simulink library "Du_Gimbal_LIB"  (R2024b)
settings: Solver=VariableStepAuto  StartTime=0.0  StopTime=10.0  RelTol=1e-3
undefined symbols (not defined in the file): Continuous, DiscIntNeverNeededParam, params, Time, Ts
libraries: arduinolib x12, fl_lib x11, nesl_utility x7, $bdroot x5, simulink x4, simulink_extras x3, MISSILE_GUIDANCE_LIB2 x3, dspstat3 x3, hdlsllib x2, ctrlSharedLib x1, ee_lib x1, arduinosensorlib x1
settings Model: Creator=leoni  LastModifiedBy=leoni

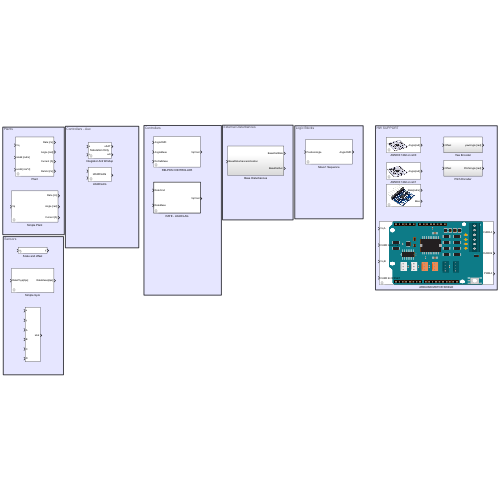
[thumbnail: Simulink's stored preview of the top-level diagram]
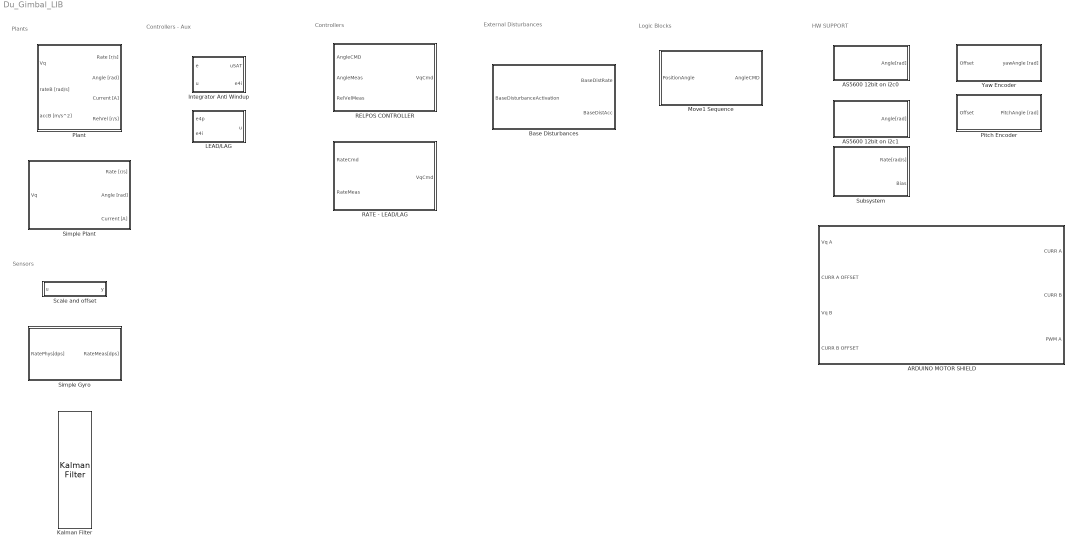
== system Du_Gimbal_LIB ==
  note: HW SUPPORT
  note: Sensors
  note: Logic Blocks
  note: Controllers
  note: Controllers - Aux
  note: Plants
  note: External Disturbances
  ARDUINO MOTOR SHIELD : Subsystem  mask{ts=1/1000, VqMax=0.85, motAdirReverse=off, motBdirReverse=off}
      mask prompts: ts "Sample Time [s]"; VqMax "Vq max."; motAdirReverse "motor A Current direction Reversed ?"; motBdirReverse "motor B Current direction Reversed ?"
      mask Display: image('arduino_motor_shield_sized_1.svg');
  AS5600 12bit on i2c0 : Subsystem  mask{deviceAddress=0x36, angleRegAddress=0x0C, ts=0.01}
      mask prompts: deviceAddress "AS 5600 Address"; angleRegAddress "Angle register"; ts "Sample Time [s]"
      mask Display: image('AS5600_ENC.png');
  AS5600 12bit on i2c1 : Subsystem  mask{deviceAddress=0x36, angleRegAddress=0x0C, ts=0.01}
      mask prompts: deviceAddress "AS 5600 Address"; angleRegAddress "Angle register"; ts "Read Time Step"
      mask Display: image('AS5600_ENC.png');
  Base Disturbances : Subsystem
  Integrator Anti Windup : Subsystem  mask{clampingOn=off, satLimit=0}
      mask prompts: clampingOn "AntiWindup Active"; satLimit "Saturation Limit"
      mask Display:
      | p = Simulink.Mask.get(gcb);
      | param = p.getParameter('clampingOn');
      | clampingOn = param.Value;
      | if contains(clampingOn,'on')
      | disp('Integrator Clamping Active');
      | else
      | disp('Saturation Only');
      | end
  Kalman Filter : ctrlSharedLib/Kalman Filter  TimeDomain=Continuous-Time  UseCurrentEstimator=on  ModelSource=Input port  ModelSourceVariable=ss(0.95,1,1,0,1)  A=0.95  B=1  C=1  D=0  NumberOfStates=1  NumberOfInputs=1  NumberOfOutputs=1  InitialEstimateSource=Dialog  X0=0  P0=10  UseK=off  UseGH=off  NumberOfProcessNoiseInputs=1  G=1  TimeInvariantG=on  H=0  TimeInvariantH=on  Q=0.05  TimeInvariantQ=on  R=1  TimeInvariantR=on  N=0  TimeInvariantN=on  AddInputPort=on  AddEnablePort=off  OutputEstimatedY=off  OutputP=off  Ts=-1
  LEAD/LAG : Subsystem  mask{isPiFlag=0, Kc=0, tau_N=0, tau_D=1.0, Ts=0}
      mask prompts: isPiFlag "is PI ?"; Kc "Controller Gain"; tau_N "Numerator Time Constant [s]"; tau_D "Denominator time Constant [s]"; Ts "Sampling Time [s]"
      mask Callback isPiFlag:
      | p = Simulink.Mask.get(gcb);
      |     param = p.getParameter('isPiFlag');
      |     slave = p.getParameter('tau_D');
      |     isPI = param.Value;
      |     if contains(isPI,'1')
      |         slave.Value = '1.0';
      |         slave.Visible = 'off';
      |     else
      |         slave.Visible = 'on';
      |     end
      mask Display:
      | p = Simulink.Mask.get(gcb);
      | param = p.getParameter('isPiFlag');
      | isPi = param.Value;
      | if contains(isPi,'1')
      | disp('PI Controller');
      | else
      | disp('LEAD/LAG');
      | end
  Move1 Sequence : Subsystem  mask{theta_dot_cmd=5, theta_travel=16, t_start=2, t_at_limit=0.5, theta_delta=1.0}
      mask prompts: theta_dot_cmd "Motion Speed [deg/s]"; theta_travel "Single Side Angle [deg]"; t_start "Start Motion Time [s]"; t_at_limit "Limit Idle Time [s]"; theta_delta "Limit Proximity Value [deg]"
      mask DialogControl ParameterGroupVar Prompt: Move1 Generator
  Pitch Encoder : Subsystem
  Plant : Subsystem  mask{L_m=1.2e-3, R_m=6.9, Kt=0.0116, V_bus=6.0, J_m=3.2e-7, J_L=200e-6, limit_DEG=17, T_r=1.8e-3, K_spr=25e-3, UNB_mag=300e-6, UNB_pos=deg2rad(45)}
      mask prompts: L_m "Inductance [H]"; R_m "Resistance [Ohm]"; Kt "Torque Constant [Nm/A]"; V_bus "Vbus [V]"; J_m "Motor Rotor Inertia [kg m^2]"; J_L "Load Inertia [kg m^2]"; limit_DEG "Travel Limit [deg]"; T_r "Friction Torque [Nm]"; K_spr "Spring Constant [Nm/Rad]"; UNB_mag "Unbalance Mag. [kg*m]"; UNB_pos "Unbalance Angle [rad]"
      mask DialogControl ParameterGroupVar Prompt: Motor Parameters
      mask DialogControl Container3 Prompt: Load Properties
      mask DialogControl Container4 Prompt: Disturbances Properties
  RATE - LEAD/LAG : Subsystem  TreatAsAtomicUnit=on  SystemSampleTime=Ts  mask{lagParams=params.LAG, leadParams=params.LEAD, VqRatioFromMAX=0.95, VqMAX=1.0}
      mask prompts: lagParams "LAG Controller Parameters"; leadParams "LEAD Controller Parameters"; VqRatioFromMAX "Vq Clamping Ratio from MAX."; VqMAX "Vq Max. CMD"
      mask DialogControl ParameterGroupVar Prompt: Controllers
      mask DialogControl Container3 Prompt: Saturations
  RELPOS CONTROLLER : Subsystem  mask{Kp=25, Kv=2.5, Vq_sat=0.95}
      mask prompts: Kp "Angle Error Gain"; Kv "Vel Error Gain"; Vq_sat "Max. Vq Cmd."
      mask DialogControl ParameterGroupVar Prompt: RELPOS CASCADE
  Scale and offset : Subsystem  mask{scale=0, offset=0}
  Simple Gyro : Subsystem  mask{scaleFactor=params.GYRO.SF_proc, a2dSens=params.GYRO.a2dSens, gyrosMA=params.GYRO.gyrosMA_proc, bias=params.GYRO.bias, biasInstability=params.GYRO.biasInstability, gSens=params.GYRO.gSens, noiseDensity=params.GYRO.noiseDensity, friqFIlter=params.GYRO.freqFilter, zetaFilter=params.GYRO.zetaFilter, dataRate=params.GYRO.dataRate, rngSeed=0}
      mask prompts: scaleFactor "Scale Factor [%]"; a2dSens "Sensetivity Scale Factor [LSB/dps]"; gyrosMA "Cross Axis Sensetivity [%]"; bias "Bias [deg/s]"; biasInstability "Time Drift [deg/s/s]"; gSens "Linear Acceleration Sensetivity"; noiseDensity "Noise Denisty [dps/sqrt_Hz]"; friqFIlter "Filter Bandwith [Hz]"; zetaFilter "Filter Zeta"; dataRate "Data Rate [Hz]"; rngSeed "RNG SEED"
      mask init:
      | rng(rngSeed);
      |     randFactors = rand(7,1)*2-1;
      mask DialogControl ParameterGroupVar Prompt: GYROSCOPE SENSETIVITY
      mask DialogControl Container4 Prompt: Gyroscope Zero Rate output
      mask DialogControl Container5 Prompt: Gyroscope Noise Performance
      mask DialogControl Container3 Prompt: FIlter Properties
      mask DialogControl Container6 Prompt: DATA RATE
  Simple Plant : Subsystem  mask{plantParams=params.PLANT}
      mask prompts: plantParams "Plant And Actuator Params"
  Subsystem : Subsystem  mask{ts=0, tInit=0}
      mask prompts: ts "Sampling Time [s]"; tInit "Initialization Time [s]"
      mask Display: image('MPU6050_ICON.svg');
  Yaw Encoder : Subsystem

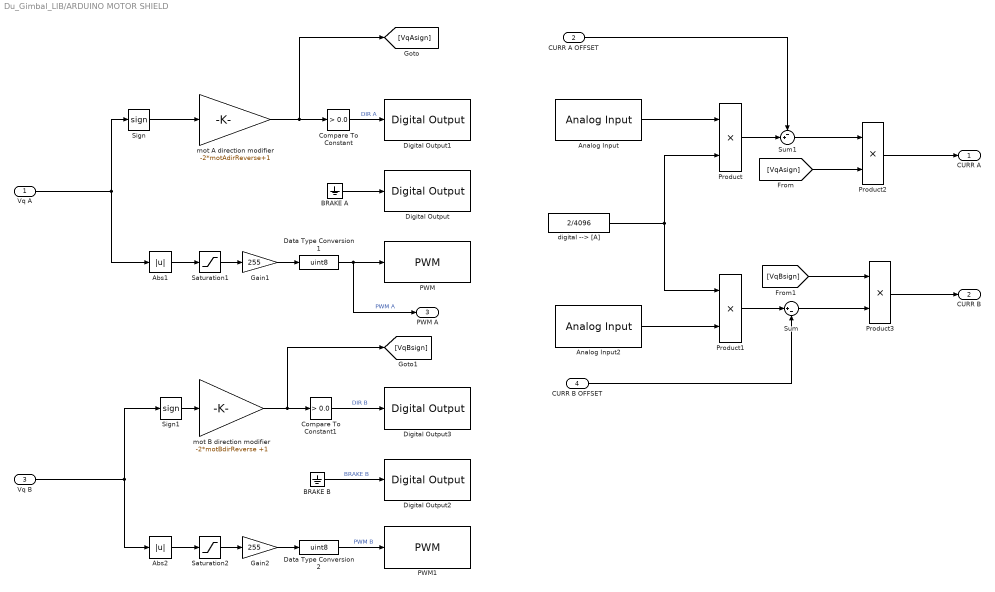
== system Du_Gimbal_LIB/ARDUINO MOTOR SHIELD ==
  Vq A : Inport
  CURR A OFFSET : Inport  Port=2
  Vq B : Inport  Port=3
  CURR B OFFSET : Inport  Port=4
  Abs1 : Abs  SaturateOnIntegerOverflow=off
  Abs2 : Abs  SaturateOnIntegerOverflow=off
  Analog Input : arduinolib/Analog Input  pinNumber=0  ReadResultsOnly=off  ConversionTriggerSource=Software  ExternalTriggerType=uint32( 0 )  OutputDataType=uint16  EnableConversionCompleteNotify=off  EnableOuputStatus=off  SampleTime=ts  blockPlatform=arduino
      settings: SourceProductName=Common
  Analog Input2 : arduinolib/Analog Input  pinNumber=1  ReadResultsOnly=off  ConversionTriggerSource=Software  ExternalTriggerType=uint32( 0 )  OutputDataType=uint16  EnableConversionCompleteNotify=off  EnableOuputStatus=off  SampleTime=ts  blockPlatform=arduino
      settings: SourceProductName=Common
  BRAKE A : Ground
  BRAKE B : Ground
  Compare To Constant : simulink/Logic and Bit Operations/Compare To Constant  relop=>  const=0.0  OutDataTypeStr=boolean
  Compare To Constant1 : simulink/Logic and Bit Operations/Compare To Constant  relop=>  const=0.0  OutDataTypeStr=boolean
  Data Type Conversion1 : DataTypeConversion  OutDataTypeStr=uint8  SaturateOnIntegerOverflow=off  RndMeth=Floor
  Data Type Conversion2 : DataTypeConversion  OutDataTypeStr=uint8  SaturateOnIntegerOverflow=off  RndMeth=Floor
  Digital Output : arduinolib/Digital Output  pinNumber=9  Direction=output  blockPlatform=arduino
      settings: SourceProductName=Common
  Digital Output1 : arduinolib/Digital Output  pinNumber=12  Direction=output  blockPlatform=arduino
      settings: SourceProductName=Common
  Digital Output2 : arduinolib/Digital Output  pinNumber=8  Direction=output  blockPlatform=arduino
      settings: SourceProductName=Common
  Digital Output3 : arduinolib/Digital Output  pinNumber=13  Direction=output  blockPlatform=arduino
      settings: SourceProductName=Common
  Gain1 : Gain  Gain=255  OutDataTypeStr=uint16
  Gain2 : Gain  Gain=255  OutDataTypeStr=uint16
  PWM : arduinolib/PWM  pinNumber=3  frequencyType=Specify  desiredFrequency=50000  achievableFrequency=490.2
      settings: SourceProductName=Common
  PWM1 : arduinolib/PWM  pinNumber=11  frequencyType=Specify  desiredFrequency=50000  achievableFrequency=490.2
      settings: SourceProductName=Common
  Product{,1..3} (4 alike) : Product
  Saturation1 : Saturate  UpperLimit=VqMax  LowerLimit=0
  Saturation2 : Saturate  UpperLimit=VqMax  LowerLimit=0
  Sign : Signum
  Sign1 : Signum
  Sum : Sum  Inputs=|+-
  Sum1 : Sum  Inputs=-+|
  digital --> [A] : Constant  Value=2/4096
  mot A direction modifier : Gain  Gain=-2*motAdirReverse+1
  mot B direction modifier : Gain  Gain=-2*motBdirReverse +1
  CURR A : Outport
  CURR B : Outport  Port=2
  PWM A : Outport  Port=3
  wires:
  BRAKE B/1 -> Digital Output2/1  "BRAKE B"
  Data Type Conversion2/1 -> PWM1/1  "PWM B"
  BRAKE A/1 -> Digital Output/1
  Data Type Conversion1/1 -> PWM A/1, PWM/1  "PWM A"
  Analog Input2/1 -> Product1/2
  Product/1 -> Sum1/2
  Product1/1 -> Sum/1
  digital --> [A]/1 -> Product/2, Product1/1
  Analog Input/1 -> Product/1
  CURR A OFFSET/1 -> Sum1/1
  Sum1/1 -> Product2/1
  Sum/1 -> Product3/2
  CURR B OFFSET/1 -> Sum/2
  Vq A/1 -> Abs1/1, Sign/1
  Abs1/1 -> Saturation1/1
  Saturation1/1 -> Gain1/1
  Gain1/1 -> Data Type Conversion1/1
  Sign1/1 -> mot B direction modifier/1
  Vq B/1 -> Sign1/1, Abs2/1
  Abs2/1 -> Saturation2/1
  Saturation2/1 -> Gain2/1
  Gain2/1 -> Data Type Conversion2/1
  Compare To Constant/1 -> Digital Output1/1  "DIR A"
  Compare To Constant1/1 -> Digital Output3/1  "DIR B"
  Product2/1 -> CURR A/1
  [VqAsign] -> Product2/2
  [VqBsign] -> Product3/1
  Product3/1 -> CURR B/1
  mot A direction modifier/1 -> [VqAsign], Compare To Constant/1
  mot B direction modifier/1 -> [VqBsign], Compare To Constant1/1
  Sign/1 -> mot A direction modifier/1

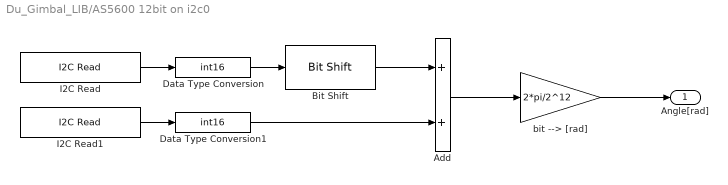
== system Du_Gimbal_LIB/AS5600 12bit on i2c0 ==
  Add : Sum
  Bit Shift : hdlsllib/Logic and Bit Operations/Bit Shift  mode=Shift Left Logical  N=8
  Data Type Conversion : DataTypeConversion  OutDataTypeStr=int16  SaturateOnIntegerOverflow=off  RndMeth=Floor
  Data Type Conversion1 : DataTypeConversion  OutDataTypeStr=int16  SaturateOnIntegerOverflow=off  RndMeth=Floor
  I2C Read : arduinolib/I2C Read  I2CModule=0  Mode=Master  SlaveAddress=deviceAddress  SlaveByteOrder=BigEndian  Direction=Receiver  RegisterAddressMode=on  RegisterAddress=angleRegAddress  SlaveDataType=uint8  DataLength=1  NoAck=off  RepeatedStart=off  OutputStatus=off  blockPlatform=ARDUINO  SampleTime=ts
      settings: SourceProductName=Common
  I2C Read1 : arduinolib/I2C Read  I2CModule=0  Mode=Master  SlaveAddress=deviceAddress  SlaveByteOrder=BigEndian  Direction=Receiver  RegisterAddressMode=on  RegisterAddress=angleRegAddress+1  SlaveDataType=uint8  DataLength=1  NoAck=off  RepeatedStart=off  OutputStatus=off  blockPlatform=ARDUINO  SampleTime=ts
      settings: SourceProductName=Common
  bit --> [rad] : Gain  Gain=2*pi/2^12
  Angle[rad] : Outport
  wires:
  Data Type Conversion1/1 -> Add/2
  Bit Shift/1 -> Add/1
  Data Type Conversion/1 -> Bit Shift/1
  I2C Read/1 -> Data Type Conversion/1
  I2C Read1/1 -> Data Type Conversion1/1
  Add/1 -> bit --> [rad]/1
  bit --> [rad]/1 -> Angle[rad]/1

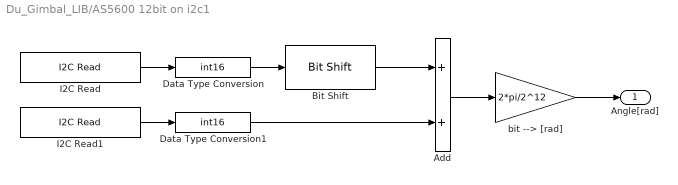
== system Du_Gimbal_LIB/AS5600 12bit on i2c1 ==
  Add : Sum
  Bit Shift : hdlsllib/Logic and Bit Operations/Bit Shift  mode=Shift Left Logical  N=8
  Data Type Conversion : DataTypeConversion  OutDataTypeStr=int16  SaturateOnIntegerOverflow=off  RndMeth=Floor
  Data Type Conversion1 : DataTypeConversion  OutDataTypeStr=int16  SaturateOnIntegerOverflow=off  RndMeth=Floor
  I2C Read : arduinolib/I2C Read  I2CModule=1  Mode=Master  SlaveAddress=deviceAddress  SlaveByteOrder=BigEndian  Direction=Receiver  RegisterAddressMode=on  RegisterAddress=angleRegAddress  SlaveDataType=uint8  DataLength=1  NoAck=off  RepeatedStart=off  OutputStatus=off  blockPlatform=ARDUINO  SampleTime=ts
      settings: SourceProductName=Common
  I2C Read1 : arduinolib/I2C Read  I2CModule=1  Mode=Master  SlaveAddress=deviceAddress  SlaveByteOrder=BigEndian  Direction=Receiver  RegisterAddressMode=on  RegisterAddress=angleRegAddress+1  SlaveDataType=uint8  DataLength=1  NoAck=off  RepeatedStart=off  OutputStatus=off  blockPlatform=ARDUINO  SampleTime=ts
      settings: SourceProductName=Common
  bit --> [rad] : Gain  Gain=2*pi/2^12
  Angle[rad] : Outport
  wires:
  Data Type Conversion1/1 -> Add/2
  Bit Shift/1 -> Add/1
  Data Type Conversion/1 -> Bit Shift/1
  I2C Read/1 -> Data Type Conversion/1
  I2C Read1/1 -> Data Type Conversion1/1
  Add/1 -> bit --> [rad]/1
  bit --> [rad]/1 -> Angle[rad]/1

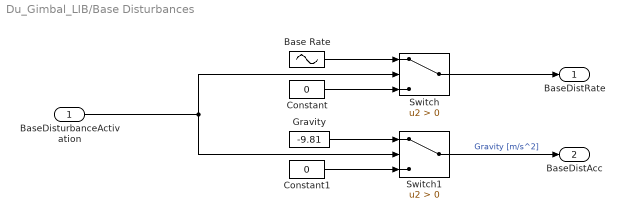
== system Du_Gimbal_LIB/Base Disturbances ==
  BaseDisturbanceActivation : Inport
  Base Rate : Sin  Amplitude=deg2rad(20)  Frequency=2*pi*2  SampleTime=0
  Constant : Constant  Value=0
  Constant1 : Constant  Value=0
  Gravity : Constant  Value=-9.81
  Switch : Switch  Criteria=u2 > Threshold  SaturateOnIntegerOverflow=off  InputSameDT=off
  Switch1 : Switch  Criteria=u2 > Threshold  SaturateOnIntegerOverflow=off  InputSameDT=off
  BaseDistRate : Outport
  BaseDistAcc : Outport  Port=2
  wires:
  BaseDisturbanceActivation/1 -> Switch1/2, Switch/2
  Constant/1 -> Switch/3
  Gravity/1 -> Switch1/1
  Base Rate/1 -> Switch/1
  Switch/1 -> BaseDistRate/1
  Constant1/1 -> Switch1/3
  Switch1/1 -> BaseDistAcc/1  "Gravity [m/s^2]"

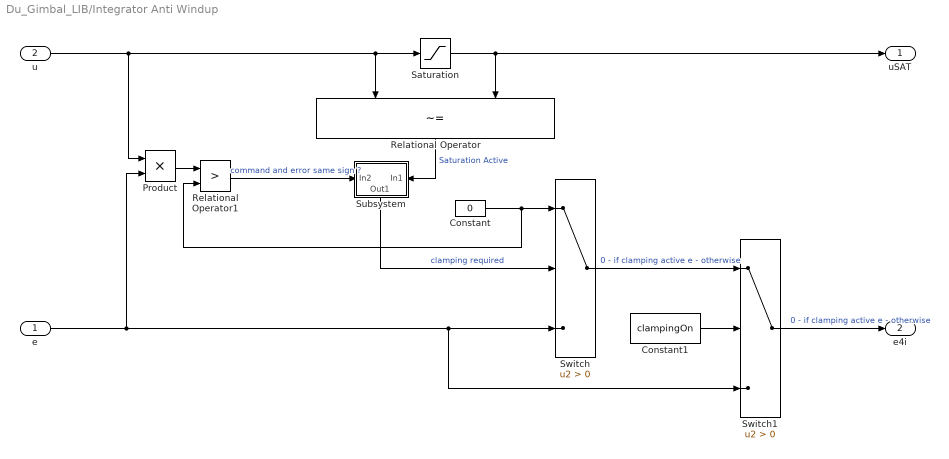
== system Du_Gimbal_LIB/Integrator Anti Windup ==
  e : Inport
  u : Inport  Port=2
  Constant : Constant  Value=0
  Constant1 : Constant  Value=clampingOn
  Product : Product
  Relational Operator : RelationalOperator  Operator=~=  OutDataTypeStr=boolean  RndMeth=Simplest  InputSameDT=off
  Relational Operator1 : RelationalOperator  Operator=>  OutDataTypeStr=boolean  RndMeth=Simplest  InputSameDT=off
  Saturation : Saturate  UpperLimit=satLimit  LowerLimit=-satLimit
  Subsystem : Subsystem
      settings: PortSchema="{\"entries\":[{\"content\":{\"sides\":[{\"content\":{},\"type\":\"ConnectorPlacement.EquallySpacedRectSide\",\"uuid\":\"a9aec0d1-7f20-4b23-b37e-cf2c45620145\"},{\"content\":{\"connectorIds\":[\"Out1\"],\"side\":\"RIGHT\"},\"type\":\"ConnectorPlacement.EquallySpacedRectSide\",\"uuid\":\"46d94b5a-ca40-426c-ab7c-6dcf988cef68\"},{\"content\":{\"connectorIds\":[\"In1\"],\"side\":\"TOP\"},\"type\":\"ConnectorPlacement.EquallySpacedRectSide\",\"uuid\":\"2dd56584-143a-41c5-aa39-bf48e1e5c5d9\"},{\"content\":{\"connectorIds\":[\"In2\"],\"side\":\"BOTTOM\"},\"type\":\"ConnectorPlacement.EquallySpacedRectSide\",\"uuid\":\"3500ab9b-abc5-4f65-b64c-eef04de61636\"}]},\"type\":\"ConnectorPlacement.EquallySpacedConnector\",\"uuid\":\"f9745eab-cd5d-404d-8705-919820576021\"}],\"packageUris\":[\"http://schema.mathworks.com/mf0/Connector/R2020b\"],\"version\":\"1.0\"}"
      mask Display: disp('AND');
  Switch : Switch  Criteria=u2 > Threshold  SaturateOnIntegerOverflow=off  InputSameDT=off
  Switch1 : Switch  Criteria=u2 > Threshold  SaturateOnIntegerOverflow=off  InputSameDT=off
  uSAT : Outport
  e4i : Outport  Port=2
  wires:
  e/1 -> Product/2, Switch1/3, Switch/3
  Subsystem/1(Out1) -> Switch/2  "clamping required"
  u/1 -> Product/1, Saturation/1, Relational Operator/1
  Saturation/1 -> uSAT/1, Relational Operator/2
  Relational Operator/1 -> Subsystem/2(In1)  "Saturation Active"
  Switch/1 -> Switch1/1  "0 - if clamping active e - otherwise"
  Constant/1 -> Relational Operator1/2, Switch/1
  Product/1 -> Relational Operator1/1
  Relational Operator1/1 -> Subsystem/1(In2)  "command and error same sign ?"
  Switch1/1 -> e4i/1  "0 - if clamping active e - otherwise"
  Constant1/1 -> Switch1/2

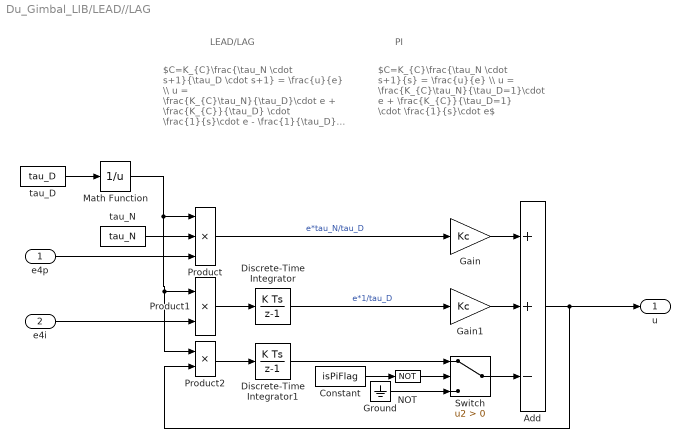
== system Du_Gimbal_LIB/LEAD//LAG ==
  note: LEAD/LAG
  note: $C=K_{C}\frac{\tau_N \cdot s+1}{\tau_D \cdot s+1} = \frac{u}{e} \\ u = \frac{K_{C}\tau_N}{\tau_D}\cdot e + \frac{K_{C}}{\tau_D} \cdot \frac{1}{s}\cdot e - \frac{1}{\tau_D} \cdot \frac{1}{s}\cdot u$
  note: PI
  note: $C=K_{C}\frac{\tau_N \cdot s+1}{s} = \frac{u}{e} \\ u = \frac{K_{C}\tau_N}{\tau_D=1}\cdot e + \frac{K_{C}}{\tau_D=1} \cdot \frac{1}{s}\cdot e$
  e4p : Inport
  e4i : Inport  Port=2
  Add : Sum  Inputs=++-
  Constant : Constant  Value=isPiFlag
  Discrete-Time Integrator : DiscreteIntegrator  SampleTime=Ts  ICPrevOutput=DiscIntNeverNeededParam  ICPrevScaledInput=DiscIntNeverNeededParam
  Discrete-Time Integrator1 : DiscreteIntegrator  SampleTime=Ts  ICPrevOutput=DiscIntNeverNeededParam  ICPrevScaledInput=DiscIntNeverNeededParam
  Gain : Gain  Gain=Kc
  Gain1 : Gain  Gain=Kc
  Ground : Ground
  Math Function : Math  Operator=reciprocal
  NOT : Logic  Operator=NOT  AllPortsSameDT=off  OutDataTypeStr=boolean
  Product : Product  Inputs=***
  Product1 : Product  Inputs=**
  Product2 : Product  Inputs=**
  Switch : Switch  Criteria=u2 > Threshold  SaturateOnIntegerOverflow=off  InputSameDT=off
  tau_D : Constant  Value=tau_D
  tau_N : Constant  Value=tau_N
  u : Outport
  wires:
  e4p/1 -> Product/3
  Add/1 -> Product2/2, u/1
  tau_D/1 -> Math Function/1
  Math Function/1 -> Product2/1, Product1/1, Product/1
  tau_N/1 -> Product/2
  Product/1 -> Gain/1  "e*tau_N/tau_D"
  Product1/1 -> Discrete-Time Integrator/1
  Discrete-Time Integrator/1 -> Gain1/1  "e*1/tau_D"
  Product2/1 -> Discrete-Time Integrator1/1
  Discrete-Time Integrator1/1 -> Switch/1
  e4i/1 -> Product1/2
  Gain/1 -> Add/1
  Gain1/1 -> Add/2
  Switch/1 -> Add/3
  Constant/1 -> NOT/1
  NOT/1 -> Switch/2
  Ground/1 -> Switch/3

== system Du_Gimbal_LIB/Move1 Sequence ==
  PositionAngle : Inport
  Degrees to Radians : simulink_extras/Transformations/Degrees to Radians
  MOVE1 LOGIC - Degrees : Stateflow chart  TreatAsAtomicUnit=on
  Radians to Degrees : simulink_extras/Transformations/Radians to Degrees
  Rate Limiter : RateLimiter  RisingSlewLimit=theta_dot_cmd  FallingSlewLimit=-theta_dot_cmd  SampleTimeMode=inherited
  AngleCMD : Outport
  wires:
  MOVE1 LOGIC - Degrees/1(PosCmd) -> Rate Limiter/1
  Degrees to Radians/1 -> AngleCMD/1
  Rate Limiter/1 -> Degrees to Radians/1
  PositionAngle/1 -> Radians to Degrees/1
  Radians to Degrees/1 -> MOVE1 LOGIC - Degrees/1(PosRtn)

== system Du_Gimbal_LIB/Pitch Encoder ==
  Offset : Inport
  AS5600 12bit on i2c1 : $bdroot/AS5600 12bit on i2c1  deviceAddress=0x36  angleRegAddress=0x0C  ts=0.01
  DirectionModifier : Gain  Gain=-1
  Sum : Sum  Inputs=|+-
  PitchAngle [rad] : Outport
  wires:
  Sum/1 -> DirectionModifier/1
  AS5600 12bit on i2c1/1 -> Sum/1
  Offset/1 -> Sum/2
  DirectionModifier/1 -> PitchAngle [rad]/1

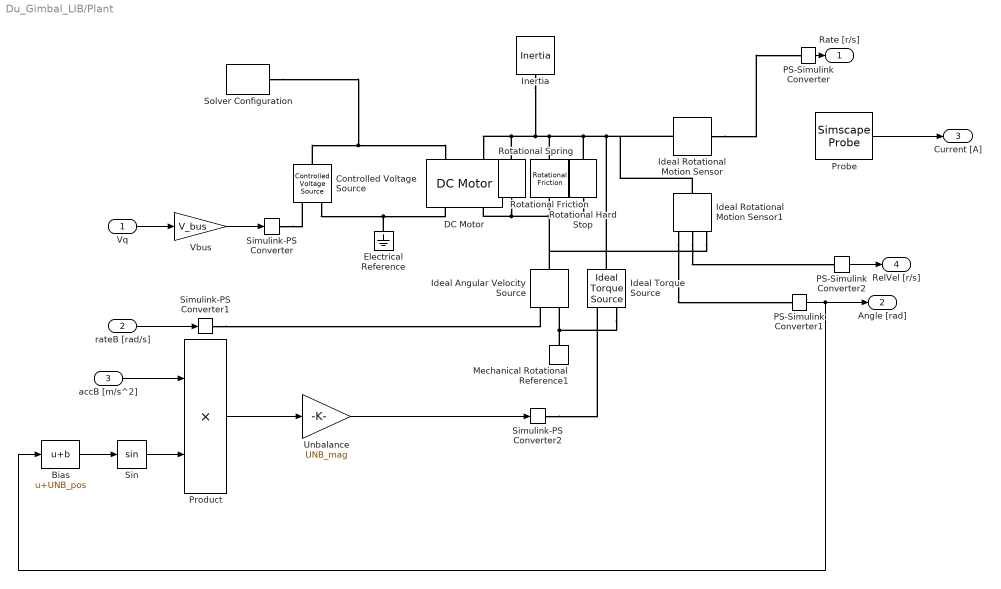
== system Du_Gimbal_LIB/Plant ==
  Vq : Inport
  rateB [rad/s] : Inport  Port=2
  accB [m/s^2] : Inport  Port=3
  Bias : Bias  Bias=UNB_pos  SaturateOnIntegerOverflow=off
  Controlled Voltage Source : fl_lib/Electrical/Electrical Sources/Controlled Voltage Source
  DC Motor : ee_lib/Electromechanical/Brushed Motors/DC Motor  field_option=ee.enum.field_option.pm  Rf=100 Ohm  Lf=1 H  Laf=0.15 H  If0=0 A  parameterization=ee.enum.dcparam_option.circuit_param  Ra=R_m Ohm  La=L_m H  emf_or_torque=ee.enum.emf_or_torque.kv  Kv=Kt V/(rad/s)  Ki=6.876e-4 N*m/A  T_stall=T_p N*m  w_max=w_NL rad/s  w_rated=15000 rpm  P_rated=0.08 W  V_rated=V_n V  lam_param=ee.enum.lam_param.damping  i_noload=0 A  V_i_noload=1.5 V  J=J_m kg*m^2  lam=0 N*m*s/rad  speed0=0 rpm  t_fault_armature=1 s  t_fault_field=1 s  fault_action=simscape.enum.assert.action.none  alpha=3.93e-3 1/K  Tmeas=25 degC  thermal_mass=100 J/K  initial_temperature=25 degC
  Electrical Reference : fl_lib/Electrical/Electrical Elements/Electrical Reference
  Ideal Angular Velocity Source : fl_lib/Mechanical/Mechanical Sources/Ideal Angular Velocity Source
  Ideal Rotational Motion Sensor : fl_lib/Mechanical/Mechanical Sensors/Ideal Rotational Motion Sensor  reference=foundation.enum.MeasurementReference.absolute  acceleration_port=false  velocity_port=true  position_port=false  wrap_angle=false  offset=0 deg
      settings: InternalSimscapePortConfiguration="{\"Bottom\":[],\"Left\":[{\"id\":\"R\",\"label\":\"R\",\"type\":\"foundation.mechanical.rotational.rotational\"}],\"Right\":[{\"id\":\"W\",\"label\":\"W\",\"type\":\"output\"}],\"Top\":[]}"
  Ideal Rotational Motion Sensor1 : fl_lib/Mechanical/Mechanical Sensors/Ideal Rotational Motion Sensor  reference=foundation.enum.MeasurementReference.difference  acceleration_port=false  velocity_port=true  position_port=true  wrap_angle=false  offset=0 rad
  Ideal Torque Source : fl_lib/Mechanical/Mechanical Sources/Ideal Torque Source
  Inertia : fl_lib/Mechanical/Rotational Elements/Inertia  inertia=J_L kg*m^2  num_ports=foundation.enum.numPorts2.one  w_specify=off  w_priority=High  w=0 rad/s  w_nominal_specify=off  w_nominal_value=1  w_nominal_unit=rad/s  t_specify=off  t_priority=None  t=0 N*m  t_nominal_specify=off  t_nominal_value=1  t_nominal_unit=N*m
  Mechanical Rotational Reference1 : fl_lib/Mechanical/Rotational Elements/Mechanical Rotational Reference
  PS-Simulink Converter : nesl_utility/PS-Simulink Converter  PhysicalDomain=network_engine_domain  SubClassName=ps_output  LeftPortType=input  RightPortType=output  PseudoPeriodic=off  Frequencies=[]  VectorFormat=inherit  Unit=inherit  AffineConversion=off
  PS-Simulink Converter1 : nesl_utility/PS-Simulink Converter  PhysicalDomain=network_engine_domain  SubClassName=ps_output  LeftPortType=input  RightPortType=output  PseudoPeriodic=off  Frequencies=[]  VectorFormat=inherit  Unit=inherit  AffineConversion=off
  PS-Simulink Converter2 : nesl_utility/PS-Simulink Converter  PhysicalDomain=network_engine_domain  SubClassName=ps_output  LeftPortType=input  RightPortType=output  PseudoPeriodic=off  Frequencies=[]  VectorFormat=inherit  Unit=inherit  AffineConversion=off
  Probe : SimscapeProbe  BoundBlock=40  Variables={i}
  Product : Product
  Rotational Friction : fl_lib/Mechanical/Rotational Elements/Rotational Friction  brkwy_trq=T_r*1.5 N*m  brkwy_vel=0.05 rad/s  Col_trq=T_r N*m  visc_coef=0 N*m*s/rad  w_specify=off  w_priority=None  w=0 rad/s  w_nominal_specify=off  w_nominal_value=1  w_nominal_unit=rad/s  t_specify=off  t_priority=None  t=0 N*m  t_nominal_specify=off  t_nominal_value=1  t_nominal_unit=N*m
  Rotational Hard Stop : fl_lib/Mechanical/Rotational Elements/Rotational Hard Stop  upper_bnd=limit_DEG deg  lower_bnd=-limit_DEG deg  model=simscape.enum.hardstop.modechart  stiff_up=1e6 N*m/rad  stiff_low=1e6 N*m/rad  D_up=0.01 N*m*s/rad  D_low=0.01 N*m*s/rad  transition=0.001 rad  coeff_rest=0.7  w_tol=0.05 rad/s  trq_tol=K_spr*deg2rad(limit_DEG) N*m  w_specify=off  w_priority=None  w=0 rad/s  w_nominal_specify=off  w_nominal_value=1  w_nominal_unit=rad/s  t_specify=off  t_priority=None  t=0 N*m  t_nominal_specify=off  t_nominal_value=1  t_nominal_unit=N*m  phi_specify=off  phi_priority=High  phi=0 rad  phi_nominal_specify=off  phi_nominal_value=1  phi_nominal_unit=rad  M_specify=off  M_priority=None  M=0
  Rotational Spring : fl_lib/Mechanical/Rotational Elements/Rotational Spring  spr_rate=K_spr N*m/rad  w_specify=off  w_priority=None  w=0 rad/s  w_nominal_specify=off  w_nominal_value=1  w_nominal_unit=rad/s  t_specify=off  t_priority=None  t=0 N*m  t_nominal_specify=off  t_nominal_value=1  t_nominal_unit=N*m  phi_specify=off  phi_priority=High  phi=0 rad  phi_nominal_specify=off  phi_nominal_value=1  phi_nominal_unit=rad
  Simulink-PS Converter : nesl_utility/Simulink-PS Converter  PhysicalDomain=network_engine_domain  SubClassName=ps_input  LeftPortType=input  RightPortType=output  PseudoPeriodic=off  Frequencies=[]  NoiseDistribution=none  NoiseParameters=[]  Unit=1  AffineConversion=off  FilteringAndDerivatives=provide  SimscapeFilterOrder=1  InputFilterTimeConstant=0.001  UdotUserProvided=0
  Simulink-PS Converter1 : nesl_utility/Simulink-PS Converter  PhysicalDomain=network_engine_domain  SubClassName=ps_input  LeftPortType=input  RightPortType=output  PseudoPeriodic=off  Frequencies=[]  NoiseDistribution=none  NoiseParameters=[]  Unit=rad/s  AffineConversion=off  FilteringAndDerivatives=filter  SimscapeFilterOrder=1  InputFilterTimeConstant=0.001  UdotUserProvided=0
  Simulink-PS Converter2 : nesl_utility/Simulink-PS Converter  PhysicalDomain=network_engine_domain  SubClassName=ps_input  LeftPortType=input  RightPortType=output  PseudoPeriodic=off  Frequencies=[]  NoiseDistribution=none  NoiseParameters=[]  Unit=N*m  AffineConversion=off  FilteringAndDerivatives=filter  SimscapeFilterOrder=1  InputFilterTimeConstant=0.001  UdotUserProvided=0
  Sin : Trigonometry
  Solver Configuration : nesl_utility/Solver Configuration  PhysicalDomain=network_engine_domain  SubClassName=solver  LeftPortType=input  RightPortType=generic  Tones=[]  Harmonics=[]  SimulateNoise=off  Profile=off  UseLocalSampling=off  EnableSwitchedLinearOptims=on  FrequencyDomain=off  UseCCode=off  RelTol=0.001  AbsTol=0.001  MinStep=1e-09  ToWorkspace=off  RevertToSquareIcSolve=off  NumHomotopyIterations=100  PhasorMode=off  PhasorModeNumHarmonics=1  ConsistencySolver=NEWTON_XTOL_AFTER_FTOL  IndexReductionMethod=DerivativeReplacement  DoDC=off  ResidualTolerance=1e-09  ConsistencyTolSource=GLOBAL  ConsistencyAbsTol=0.001  ConsistencyRelTol=0.001  ConsistencyTolFactor=0.001  UseLocalSolver=off  LocalSolverChoice=NE_BACKWARD_EULER_ADVANCER  ResolveIndetEquations=on  FunctionEvalNumThread=1  LocalSolverSampleTime=0.001  DoFixedCost=off  MaxNonlinIter=3  MaxModeIter=2  ComputeImpulses=off  ImpulseIterations=2  LinearAlgebra=auto  LinearAlgebraNumThread=0  EquationFormulation=NE_TIME_EF  DelaysMemoryBudget=1024  AutomaticFiltering=on  FilteringTimeConstant=0.001  PartitionStorageMethod=AS_NEEDED  PartitionMemoryBudget=1024  PartitionMethod=ROBUST  MultibodyUseLocalSolver=off  MultibodyLocalSolverChoice=ODE1  MultibodyLocalSolverSampleTime=0.001
  Unbalance : Gain  Gain=UNB_mag
  Vbus : Gain  Gain=V_bus
  Rate [r/s] : Outport
  Angle [rad] : Outport  Port=2
  Current [A] : Outport  Port=3
  RelVel [r/s] : Outport  Port=4
  wires:
  PS-Simulink Converter/1 -> Rate [r/s]/1
  PS-Simulink Converter1/1 -> Bias/1, Angle [rad]/1
  Probe/1 -> Current [A]/1
  rateB [rad/s]/1 -> Simulink-PS Converter1/1
  accB [m/s^2]/1 -> Product/1
  Bias/1 -> Sin/1
  Sin/1 -> Product/2
  Product/1 -> Unbalance/1
  PS-Simulink Converter2/1 -> RelVel [r/s]/1
  Unbalance/1 -> Simulink-PS Converter2/1
  Vq/1 -> Vbus/1
  Vbus/1 -> Simulink-PS Converter/1
  connections:
  Controlled Voltage Source/RConn2 -- Electrical Reference/LConn1 -- DC Motor/RConn1
  Controlled Voltage Source/LConn1 -- Solver Configuration/RConn1 -- DC Motor/LConn1
  Rotational Hard Stop/LConn1 -- Ideal Torque Source/LConn1 -- Ideal Rotational Motion Sensor1/LConn1 -- Ideal Rotational Motion Sensor/LConn1 -- Rotational Spring/LConn1 -- DC Motor/LConn2 -- Inertia/LConn1 -- Rotational Friction/LConn1
  Ideal Rotational Motion Sensor/RConn1 -- PS-Simulink Converter/LConn1
  Ideal Rotational Motion Sensor1/RConn3 -- PS-Simulink Converter1/LConn1
  Rotational Hard Stop/RConn1 -- Ideal Rotational Motion Sensor1/RConn1 -- Ideal Angular Velocity Source/LConn1 -- Rotational Spring/RConn1 -- DC Motor/RConn2 -- Rotational Friction/RConn1
  Simulink-PS Converter/RConn1 -- Controlled Voltage Source/RConn1
  Mechanical Rotational Reference1/LConn1 -- Ideal Torque Source/RConn2 -- Ideal Angular Velocity Source/RConn2
  Simulink-PS Converter1/RConn1 -- Ideal Angular Velocity Source/RConn1
  Simulink-PS Converter2/RConn1 -- Ideal Torque Source/RConn1
  Ideal Rotational Motion Sensor1/RConn2 -- PS-Simulink Converter2/LConn1

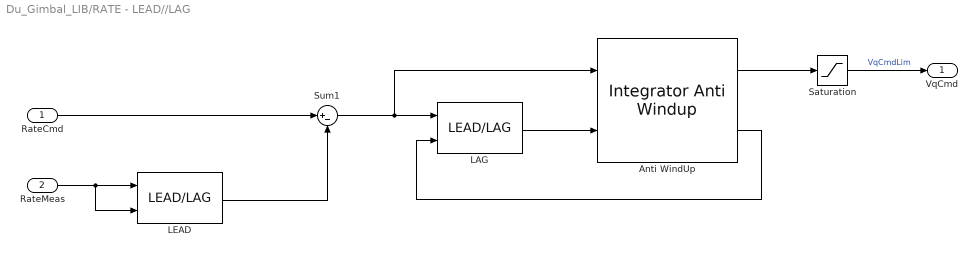
== system Du_Gimbal_LIB/RATE - LEAD//LAG ==
  RateCmd : Inport
  RateMeas : Inport  Port=2
  Anti WindUp : $bdroot/Integrator Anti Windup  clampingOn=on  satLimit=VqMAX*VqRatioFromMAX
  LAG : $bdroot/LEAD//LAG  isPiFlag=lagParams.isPiFlag  Kc=lagParams.K  tau_N=lagParams.tau_N  tau_D=1.0  Ts=Ts
  LEAD : $bdroot/LEAD//LAG  isPiFlag=leadParams.isPiFlag  Kc=leadParams.K  tau_N=leadParams.tau_N  tau_D=leadParams.tau_D  Ts=Ts
  Saturation : Saturate  UpperLimit=VqMAX  LowerLimit=-VqMAX
  Sum1 : Sum  Inputs=|+-
  VqCmd : Outport
  wires:
  LEAD/1 -> Sum1/2
  RateCmd/1 -> Sum1/1
  RateMeas/1 -> LEAD/2, LEAD/1
  Saturation/1 -> VqCmd/1  "VqCmdLim"
  Sum1/1 -> Anti WindUp/1, LAG/1
  LAG/1 -> Anti WindUp/2
  Anti WindUp/1 -> Saturation/1
  Anti WindUp/2 -> LAG/2

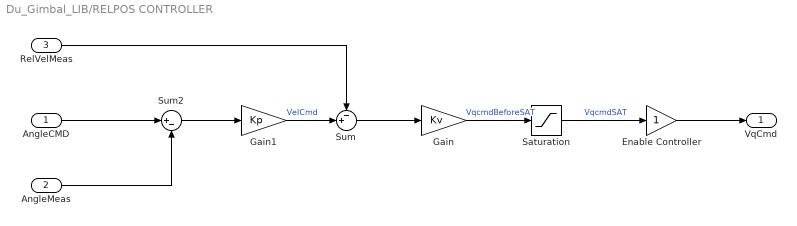
== system Du_Gimbal_LIB/RELPOS CONTROLLER ==
  AngleCMD : Inport
  AngleMeas : Inport  Port=2
  RelVelMeas : Inport  Port=3
  Enable Controller : Gain
  Gain : Gain  Gain=Kv
  Gain1 : Gain  Gain=Kp
  Saturation : Saturate  UpperLimit=Vq_sat  LowerLimit=-Vq_sat
  Sum : Sum  Inputs=-+|
  Sum2 : Sum  Inputs=|+-
  VqCmd : Outport
  wires:
  RelVelMeas/1 -> Sum/1
  Enable Controller/1 -> VqCmd/1
  Gain/1 -> Saturation/1  "VqcmdBeforeSAT"
  Sum/1 -> Gain/1
  AngleMeas/1 -> Sum2/2
  AngleCMD/1 -> Sum2/1
  Sum2/1 -> Gain1/1
  Gain1/1 -> Sum/2  "VelCmd"
  Saturation/1 -> Enable Controller/1  "VqcmdSAT"

== system Du_Gimbal_LIB/Scale and offset ==
  u : Inport
  Bias : Bias  Bias=offset  SaturateOnIntegerOverflow=off
  Gain : Gain  Gain=scale
  y : Outport
  wires:
  u/1 -> Gain/1
  Bias/1 -> y/1
  Gain/1 -> Bias/1

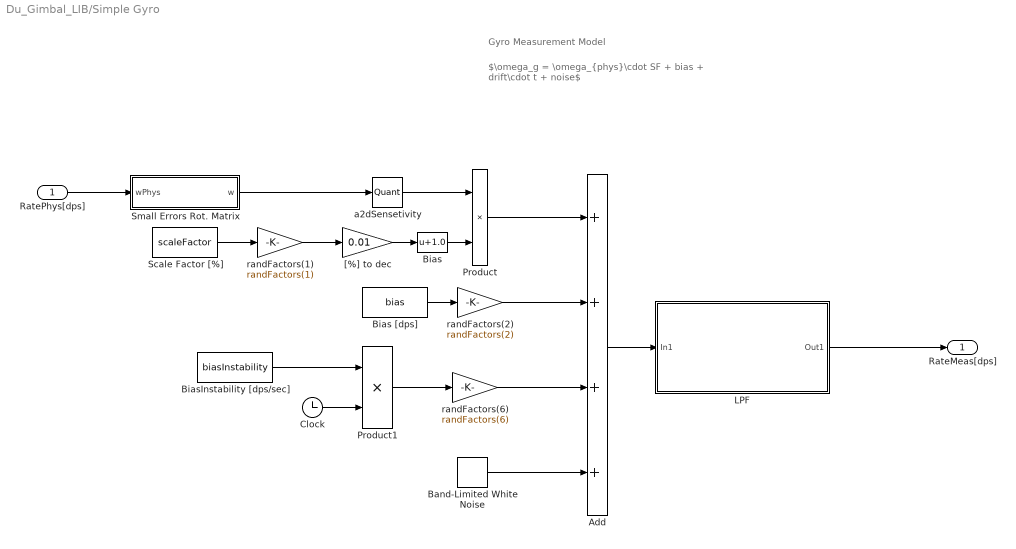
== system Du_Gimbal_LIB/Simple Gyro ==
  note: Gyro Measurement Model
  note: $\omega_g = \omega_{phys}\cdot SF + bias + drift\cdot t + noise$
  RatePhys[dps] : Inport
  Add : Sum  Inputs=++++
  Band-Limited White Noise : simulink/Sources/Band-Limited White Noise  Cov=[noiseDensity^2]  Ts=0.1  seed=[23341]
  Bias : Bias  Bias=1.0  SaturateOnIntegerOverflow=off
  Bias [dps] : Constant  Value=bias
  BiasInstability [dps/sec] : Constant  Value=biasInstability
  Clock : Clock
  LPF : Subsystem
  Product : Product
  Product1 : Product
  Scale Factor [%] : Constant  Value=scaleFactor
  Small Errors Rot. Matrix : Subsystem
  "[%] to dec" : Gain  Gain=0.01
  a2dSensetivity : Quantizer  QuantizationInterval=1/a2dSens
  randFactors(1) : Gain  Gain=randFactors(1)
  randFactors(2) : Gain  Gain=randFactors(2)
  randFactors(6) : Gain  Gain=randFactors(6)
  RateMeas[dps] : Outport  PortDimensions=[3,1]  SampleTime=1/dataRate
  wires:
  RatePhys[dps]/1 -> Small Errors Rot. Matrix/1(wPhys)
  Scale Factor [%]/1 -> randFactors(1)/1
  "[%] to dec"/1 -> Bias/1
  Product/1 -> Add/1
  a2dSensetivity/1 -> Product/1
  randFactors(1)/1 -> "[%] to dec"/1
  Bias [dps]/1 -> randFactors(2)/1
  randFactors(2)/1 -> Add/2
  Small Errors Rot. Matrix/1(w) -> a2dSensetivity/1
  Band-Limited White Noise/1 -> Add/4
  BiasInstability [dps/sec]/1 -> Product1/1
  randFactors(6)/1 -> Add/3
  Clock/1 -> Product1/2
  Product1/1 -> randFactors(6)/1
  Add/1 -> LPF/1(In1)
  LPF/1(Out1) -> RateMeas[dps]/1
  Bias/1 -> Product/2

== system Du_Gimbal_LIB/Simple Plant ==
  Vq : Inport
  Inertia : TransferFcn  Denominator=[plantParams.J 0]
  Integrator : Integrator
  Kt : Gain  Gain=plantParams.Kt
  V --> I : Gain  Gain=plantParams.Vbus/plantParams.R
  Rate [r/s] : Outport
  Angle [rad] : Outport  Port=2
  Current [A] : Outport  Port=3
  wires:
  Vq/1 -> V --> I/1  "VqCMD"
  V --> I/1 -> Current [A]/1, Kt/1  "IqCMD"
  Kt/1 -> Inertia/1  "Torque"
  Inertia/1 -> Integrator/1, Rate [r/s]/1
  Integrator/1 -> Angle [rad]/1

== system Du_Gimbal_LIB/Subsystem ==
  Bias Estimator : Subsystem  TreatAsAtomicUnit=on
  Clock : Clock
  Compare To Constant : simulink/Logic and Bit Operations/Compare To Constant  relop=<=  const=tInit  OutDataTypeStr=boolean
  Degrees to Radians2 : simulink_extras/Transformations/Degrees to Radians
  MPU6050 IMU Sensor : arduinosensorlib/MPU6050 IMU Sensor  I2CModule=0  SlaveAddress=0x68  Accel=off  AngularRate=on  Temperature=off  Status=off  Timestamp=off  EulerAngles=off  Quat=off  AccelRange=2G  GyroRange=250 dps  DmpOdr=200 Hz  Dlpf=Accelerometer: 94Hz, Gyroscope: 98Hz  spf=1  SampleTime=ts  QueueSizeFactor=1
      settings: SourceProductName=Sensors
  Sum : Sum  Inputs=|+-
  Rate[rad/s] : Outport
  Bias : Outport  Port=2
  wires:
  Clock/1 -> Compare To Constant/1
  Compare To Constant/1 -> Bias Estimator/Enable
  MPU6050 IMU Sensor/1 -> Degrees to Radians2/1
  Sum/1 -> Rate[rad/s]/1
  Bias Estimator/1(Bias) -> Bias/1, Sum/2
  Degrees to Radians2/1 -> Sum/1, Bias Estimator/1(rawGyro)

== system Du_Gimbal_LIB/Yaw Encoder ==
  Offset : Inport
  AS5600 12bit on i2c0 : $bdroot/AS5600 12bit on i2c0  deviceAddress=0x36  angleRegAddress=0x0C  ts=0.01
  Gain : Gain  Gain=-1
  Sum : Sum  Inputs=|+-
  yawAngle [rad] : Outport
  wires:
  Offset/1 -> Sum/2
  AS5600 12bit on i2c0/1 -> Sum/1
  Sum/1 -> Gain/1
  Gain/1 -> yawAngle [rad]/1

== system Du_Gimbal_LIB/Integrator Anti Windup/Subsystem ==
  In2 : Inport
  In1 : Inport  Port=2
  AND : Logic  AllPortsSameDT=off  OutDataTypeStr=boolean
  Out1 : Outport
  wires:
  In1/1 -> AND/1
  AND/1 -> Out1/1
  In2/1 -> AND/2

== system Du_Gimbal_LIB/Simple Gyro/LPF ==
  In1 : Inport
  Demux : Demux  Outputs=3
  LPF Filter : TransferFcn  Numerator=(friqFIlter*2*pi)^2  Denominator=[1 2*zetaFilter*(friqFIlter*2*pi) (friqFIlter*2*pi)^2]
  LPF Filter1 : TransferFcn  Numerator=(friqFIlter*2*pi)^2  Denominator=[1 2*zetaFilter*(friqFIlter*2*pi) (friqFIlter*2*pi)^2]
  LPF Filter2 : TransferFcn  Numerator=(friqFIlter*2*pi)^2  Denominator=[1 2*zetaFilter*(friqFIlter*2*pi) (friqFIlter*2*pi)^2]
  Mux : Mux  Inputs=3
  Out1 : Outport
  wires:
  Demux/3 -> LPF Filter2/1
  LPF Filter/1 -> Mux/1
  Demux/2 -> LPF Filter1/1
  Demux/1 -> LPF Filter/1
  LPF Filter2/1 -> Mux/3
  LPF Filter1/1 -> Mux/2
  In1/1 -> Demux/1
  Mux/1 -> Out1/1

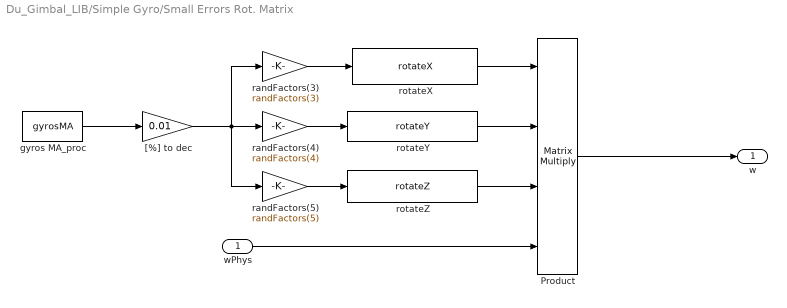
== system Du_Gimbal_LIB/Simple Gyro/Small Errors Rot. Matrix ==
  wPhys : Inport
  Product : Product  Inputs=4  Multiplication=Matrix(*)
  "[%] to dec" : Gain  Gain=0.01
  gyros MA_proc : Constant  Value=gyrosMA
  randFactors(3) : Gain  Gain=randFactors(3)
  randFactors(4) : Gain  Gain=randFactors(4)
  randFactors(5) : Gain  Gain=randFactors(5)
  rotateX : MISSILE_GUIDANCE_LIB2/rotateX  SystemSampleTime=-1  VariantActivationTime=update diagram  AllowFlexibleInterface=on  Latency=0  AutoFrameSizeCalculation=off
  rotateY : MISSILE_GUIDANCE_LIB2/rotateY  SystemSampleTime=-1  VariantActivationTime=update diagram  AllowFlexibleInterface=on  Latency=0  AutoFrameSizeCalculation=off
  rotateZ : MISSILE_GUIDANCE_LIB2/rotateZ  SystemSampleTime=-1  VariantActivationTime=update diagram  AllowFlexibleInterface=on  Latency=0  AutoFrameSizeCalculation=off
  w : Outport
  wires:
  wPhys/1 -> Product/4
  rotateZ/1 -> Product/3
  rotateY/1 -> Product/2
  rotateX/1 -> Product/1
  Product/1 -> w/1
  gyros MA_proc/1 -> "[%] to dec"/1
  randFactors(5)/1 -> rotateZ/1
  randFactors(4)/1 -> rotateY/1
  randFactors(3)/1 -> rotateX/1
  "[%] to dec"/1 -> randFactors(4)/1, randFactors(5)/1, randFactors(3)/1

== system Du_Gimbal_LIB/Subsystem/Bias Estimator ==
  rawGyro : Inport
  Enable : EnablePort  StatesWhenEnabling=reset
  Demux : Demux  Outputs=3
  Moving Average : dspstat3/Moving Average  Method=Exponential weighting  ForgettingFactorPort=off  SpecifyWindowLength=on  WindowLength=4  OverlapLength=3  AllowArbitraryInputLength=off  ForgettingFactor=0.9  SimulateUsing=Interpreted execution
  Moving Average1 : dspstat3/Moving Average  Method=Exponential weighting  ForgettingFactorPort=off  SpecifyWindowLength=on  WindowLength=4  OverlapLength=3  AllowArbitraryInputLength=off  ForgettingFactor=0.9  SimulateUsing=Interpreted execution
  Moving Average2 : dspstat3/Moving Average  Method=Exponential weighting  ForgettingFactorPort=off  SpecifyWindowLength=on  WindowLength=4  OverlapLength=3  AllowArbitraryInputLength=off  ForgettingFactor=0.9  SimulateUsing=Interpreted execution
  Vector Concatenate : Concatenate  NumInputs=3  Mode=Multidimensional array
  Bias : Outport
  wires:
  rawGyro/1 -> Demux/1
  Moving Average/1 -> Vector Concatenate/2
  Demux/1 -> Moving Average1/1
  Demux/2 -> Moving Average/1
  Demux/3 -> Moving Average2/1
  Moving Average2/1 -> Vector Concatenate/3
  Moving Average1/1 -> Vector Concatenate/1
  Vector Concatenate/1 -> Bias/1

== stateflow chart Du_Gimbal_LIB/Move1 Sequence/MOVE1 LOGIC - Degrees ==
  state IdleUntilStart
    en:
    PosCmd = PosRtn;
    ex:
    upperLimitReached = false;
    lowerLimitreached = false;
  state MovingToUpperLimit
    en:
    PosCmd = theta_travel;
    ex:
    upperLimitReached = true;
  state MovingToLowerLimit
    en:
    PosCmd = -theta_travel;
    ex:
    lowerLimitreached = true;
  state PushOnLimit
  state Completed
    en:
    PosCmd = PosRtn;
  state MovingToZero
    en:
    PosCmd = 0;
  (default) -> IdleUntilStart
  IdleUntilStart -> MovingToUpperLimit : after(t_start, sec)
  MovingToUpperLimit -> PushOnLimit : [PosRtn >= PosCmd-theta_delta]
  PushOnLimit -> MovingToLowerLimit [order 1] : after(t_at_limit,sec)[~lowerLimitreached]
  MovingToLowerLimit -> PushOnLimit : [PosRtn <= PosCmd+theta_delta]
  PushOnLimit -> MovingToZero [order 2] : after(t_at_limit,sec)
  MovingToZero -> Completed : [PosRtn >= PosCmd]
  data: t_start parameter; PosRtn input; theta_travel parameter; t_at_limit parameter; theta_delta parameter; PosCmd output; lowerLimitreached local; upperLimitReached local
